simulink model "MPC_Simulated"  (R2023a)
settings: Solver=ode1  StartTime=0.0  StopTime=360  FixedStep=1  RelTol=1e-3
values from neighbouring files (symbols this model uses):
  A = dsys.A    [CasadiSetup.m]
  B = dsys.B    [CasadiSetup.m]
  C = dsys.C    [CasadiSetup.m]
  D = 0    [CasadiSetup.m]
  m = 1    [CasadiSetup.m]    (also in CasadiSolver.m = size(du,1))
  N = 3    [CasadiSetup.m]    (also in CasadiSolver.m = size(x,2))
  n = 2    [CasadiSetup.m]    (also in CasadiSolver.m = size(x,1))
  p = 1    [CasadiSetup.m]
undefined symbols (not defined in the file or in its folder): CasadiSolver
libraries: simulink x2
settings Model: Creator=Christian  LastModifiedBy=Christian

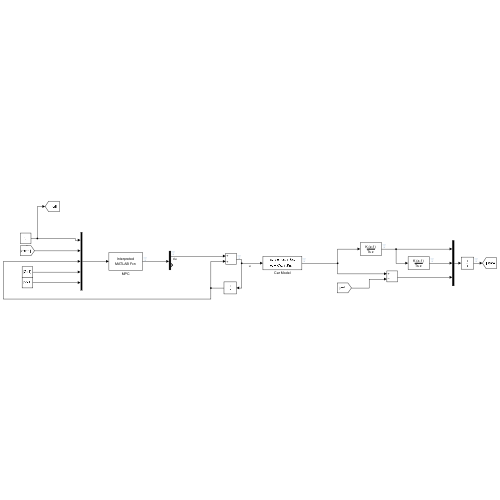
[thumbnail: Simulink's stored preview of the top-level diagram]
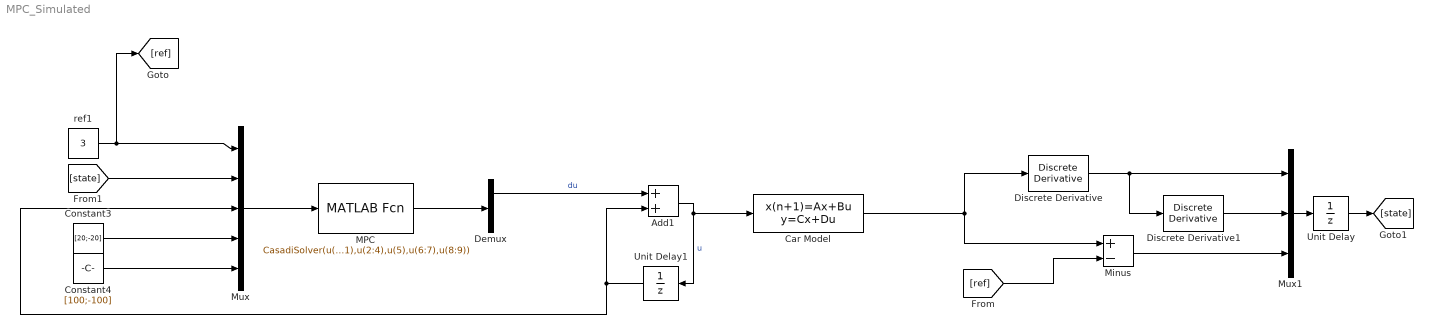
== system MPC_Simulated ==
  Add1 : Sum
  Car Model : DiscreteStateSpace  A=A  B=B  C=C  D=D
  Constant3 : Constant  Value=[20;-20]
  Constant4 : Constant  Value=[100;-100]
  Demux : Demux  Outputs=2
  Discrete Derivative : simulink/Discrete/Discrete Derivative  gainval=1.0  ICPrevScaledInput=0.0  OutMin=[]  OutMax=[]  OutDataType=fixdt(1, 16)  OutScaling=2^-10  DoSatur=off
  Discrete Derivative1 : simulink/Discrete/Discrete Derivative  gainval=1.0  ICPrevScaledInput=0.0  OutMin=[]  OutMax=[]  OutDataType=fixdt(1, 16)  OutScaling=2^-10  DoSatur=off
  MPC : MATLABFcn  MATLABFcn=CasadiSolver(u(1),u(2:4),u(5),u(6:7),u(8:9))  OutputDimensions=[1,(N*m+N*(n+p))]  Output1D=off
  Minus : Sum  Inputs=+-
  Mux : Mux  Inputs=5
  Mux1 : Mux  Inputs=3
  Unit Delay : UnitDelay  SampleTime=-1  HasFrameUpgradeWarning=on
  Unit Delay1 : UnitDelay  SampleTime=-1  HasFrameUpgradeWarning=on
  ref1 : Constant  Value=3
  wires:
  Car Model/1 -> Discrete Derivative/1, Minus/1
  Mux/1 -> MPC/1
  [state] -> Mux/2
  Constant3/1 -> Mux/4
  Unit Delay1/1 -> Mux/3, Add1/2
  Constant4/1 -> Mux/5
  MPC/1 -> Demux/1
  Add1/1 -> Car Model/1, Unit Delay1/1  "u"
  Discrete Derivative/1 -> Mux1/1, Discrete Derivative1/1
  Discrete Derivative1/1 -> Mux1/2
  Minus/1 -> Mux1/3
  ref1/1 -> Mux/1, [ref]
  [ref] -> Minus/2
  Mux1/1 -> Unit Delay/1
  Unit Delay/1 -> [state]
  Demux/1 -> Add1/1  "du"
